simulink model "Yaw_Actuation_Testrig_org"  (Simulink 10.0)
settings: Solver=ode15s  StartTime=0.0  StopTime=40  RelTol=1e-3  EnableMultiTasking=on
undefined symbols (not defined in the file): sigbuilder_block, WT_Params
libraries: fl_lib x6, nesl_utility x3, Yaw_Motor_Lib x1, Yaw_Gearbox_Lib x1
Description:
  | Copyright 2009-2017 The MathWorks, Inc. MathWorks, Inc.
settings Model: Creator=smiller  LastModifiedBy=bhisma
settings DataIOCC: LimitDataPoints=on  SignalLoggingSaveFormat=ModelDataLogs
settings OptimizationCC: ExpressionDepthLimit=2147483647
settings DebuggingCC: FcnCallInpInsideContextMsg=warning  AllowSymbolicDim=off  StateNameClashWarn=warning
settings GRTTargetCC: GeneratePreprocessorConditionals=Disable all
settings ConfigComp: CovExternalEMLEnable=off  CovSFcnEnable=off
settings SimscapeCC: SimscapeNormalizeSystem=off  SimscapeNominalValues="[{\"value\":\"10\",\"unit\":\"V\"},{\"value\":\"1\",\"unit\":\"A\"},{\"value\":\"10\",\"unit\":\"N*m\"},{\"value\":\"10\",\"unit\":\"bar\"},{\"value\":\"100\",\"unit\":\"kJ/kg\"},{\"value\":\"1\",\"unit\":\"kW\"},{\"value\":\"300\",\"unit\":\"K\"},{\"value\":\"100\",\"unit\":\"cm^3/s\"},{\"value\":\"1\",\"unit\":\"kN\"},{\"value\":\"1\",\"unit\":\"g/cm^3\"},{\"value\":\"1\",\"unit\":\"l\"},{\"value\":\"1\",\"unit\":\"cm^2\"},{\"value\":\"60\",\"unit\":\"Hz\"}]"

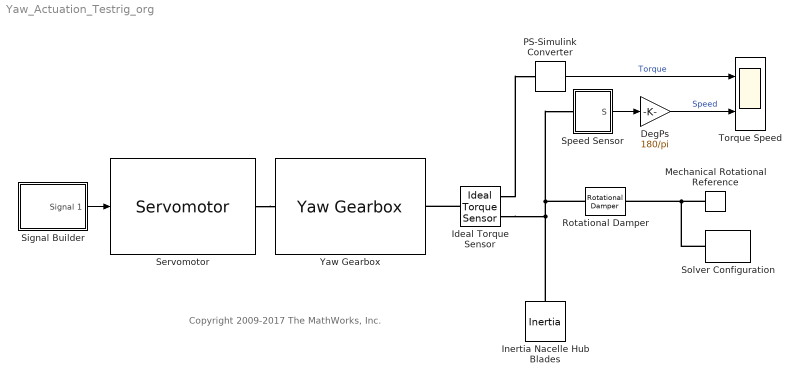
== system Yaw_Actuation_Testrig_org ==
  note: Copyright 2009-2017 The MathWorks, Inc.
  DegPs : Gain  Gain=180/pi
  Ideal Torque Sensor : fl_lib/Mechanical/Mechanical Sensors/Ideal Torque Sensor
  Inertia Nacelle Hub Blades : fl_lib/Mechanical/Rotational Elements/Inertia  inertia=WT_Params.Nacelle.inertia(1,1)*10 kg*m^2  w_specify=on  w_priority=High  w=0 rad/s  w_nominal_specify=off  w_nominal_unit=rad/s  w_nominal_value=1  t_specify=off  t_priority=High  t=0 N*m  t_nominal_specify=off  t_nominal_unit=N*m  t_nominal_value=1
  Mechanical Rotational Reference : fl_lib/Mechanical/Rotational Elements/Mechanical Rotational Reference
  PS-Simulink Converter : nesl_utility/PS-Simulink Converter  PhysicalDomain=network_engine_domain  SubClassName=ps_output  LeftPortType=input  RightPortType=output  PseudoPeriodic=off  Frequencies=[]  Unit=1  AffineConversion=off
  Rotational Damper : fl_lib/Mechanical/Rotational Elements/Rotational Damper  D=WT_Params.Nacelle.damping/4 N*m/(rad/s)  w_specify=off  w_priority=High  w=0 rad/s  w_nominal_specify=off  w_nominal_unit=rad/s  w_nominal_value=1  t_specify=off  t_priority=High  t=0 N*m  t_nominal_specify=off  t_nominal_unit=N*m  t_nominal_value=1
  Servomotor : Yaw_Motor_Lib/Yaw Motor/Servomotor  SystemSampleTime=-1
  Signal Builder : Subsystem  Tag=STV Subsys  LoadFcn=sigbuilder_block('load');  StartFcn=sigbuilder_block('start');  StopFcn=sigbuilder_block('stop');  ClipboardFcn=sigbuilder_block('clipboard');  mask(Sigbuilder block){tuvar=[0:10]}
      mask help: Create and generate interchangeable groups of signals whose waveforms are piecewise linear.
      mask init:
      | if ~strcmp(get_param(bdroot(gcbh),'SimulationStatus'),'stopped') tuvar = sigbuilder_block('maskInit'); end
      settings: CopyFcn=sigbuilder_block('copy');  DeleteFcn=sigbuilder_block('delete');  ModelCloseFcn=sigbuilder_block('modelClose');  PreSaveFcn=sigbuilder_block('preSave');  PauseFcn=sigbuilder_block('pause')  ContinueFcn=sigbuilder_block('continue')  NameChangeFcn=sigbuilder_block('namechange');  OpenFcn=sigbuilder_block('open',[437.25 199.5 550.5 399.75 ]);  CloseFcn=sigbuilder_block('close');
      mask Display: plot(0, 0, 100, 100,[2, 2, 32, 32, 2], [68, 8, 8, 68, 68],[32, 2], [38, 38], [32, 19, 2],[53, 60, 44], [32, 17, 17, 2],[16, 16, 31, 31]);txt = getActiveGroup(gcbh);text(2, 100, txt,'verticalAlignment', 'top');
  Solver Configuration : nesl_utility/Solver Configuration  PhysicalDomain=network_engine_domain  SubClassName=solver  LeftPortType=input  RightPortType=generic  Tones=[]  Harmonics=[]  SimulateNoise=off  Profile=off  UseLocalSampling=off  EnableSwitchedLinearOptims=on  FrequencyDomain=off  UseCCode=off  RelTol=0.001  AbsTol=1e-06  MinStep=1e-09  ToWorkspace=off  RevertToSquareIcSolve=off  NumHomotopyIterations=100  PhasorMode=off  PhasorModeNumHarmonics=1  DoDC=off  ResidualTolerance=1e-9  UseLocalSolver=off  LocalSolverChoice=NE_BACKWARD_EULER_ADVANCER  LocalSolverSampleTime=.001  DoFixedCost=off  MaxNonlinIter=3  MaxModeIter=2  LinearAlgebra=Sparse  EquationFormulation=NE_TIME_EF  DelaysMemoryBudget=1024  AutomaticFiltering=on  FilteringTimeConstant=0.001  PartitionStorageMethod=AS_NEEDED  PartitionMemoryBudget=1024  PartitionMethod=FAST
  Speed Sensor : Subsystem
      mask Display:
      | plot([149.600878633536;150.016472378793;150.47508104106;150.972287968219;151.50330478576;152.063017511447;152.646035805762;153.246744883819;153.859359588817;154.477980106257;155.096648782383;155.709407499646;156.310355056631;156.893703999851;157.453836360095;157.985357756531;158.483149347555;158.942417128023;159.358738098149;159.728102859405;160.046954227227;160.312221488639;160.521349974904;160.672325664379;160.763694578642;160.794576785101;160.764674871227;160.674276808796;160.524253180566;160.316048796087;160.051668777399;159.733659248606;159.365082815313;158.949489070056;158.490880407788;157.993673480629;157.462656663088;156.908284800231], [156.971389291536;157.430657072004;157.84697804213;158.216342803387;158.535194171208;158.80046143262;159.009589918885;159.16056560836;159.251934522623;159.282816729083;159.252914815208;159.162516752777;159.012493124547;158.804288740068;158.53990872138;158.221899192587;157.853322759294;157.437729014037;156.979120351769;156.48191342461;155.950896607069;155.391183881382;154.808165587067;154.20745650901;153.594841804012;152.976221286573;152.357552610446;151.744793893183;151.143846336199;150.560497392978;150.000365032735;149.468843636298;148.971052045274;148.511784264806;148.095463294681;147.726098533424;147.407247165603;147.144199990631])
      | plot([152.057635404444;152.93604260309;153.834625296826;154.744729643097;155.657590839533;156.564417533794;157.45647648909;158.325176690034;159.162152078811;159.959342124889;160.709069452336;161.404113777147;162.037781442523;162.603969882449;163.097226392739;163.512800643557;163.846690427691;164.095680203997;164.257372064819;164.330208829146;164.313489039122;164.27939575172], [142.228020686971;141.979030910664;141.817339049842;141.744502285515;141.761222075539;141.867337399197;142.061826307913;142.342815767178;142.707599694895;143.152665022428;143.673725527376;144.265763112236;144.923076131425;145.639334301243;146.40763966397;147.220593018964;148.070365181011;148.948772379657;149.847355073393;150.757459419663;151.6703206161;152.055850472277])
      | plot([116.468514315784;116.438789536125;116.349901463023;116.202706137216;115.998621130155;115.739611892022;115.42817282337;115.067303252679;114.660478551187;114.211616663162;113.725040373958;113.205435679231;112.657806656235;112.087427271827;111.499790591278;110.900555877058;110.29549408704;109.690432297022;109.091197582803;108.503560902254;107.933181517846;107.38555249485;106.865947800123;106.379371510919;105.930509622894;105.523684921402;105.162815350711;104.851376282059;104.592367043926;104.388282036865;104.241086711057;104.152198637956;104.122473858297;104.152198637956;104.241086711057;104.388282036865;104.592367043926;104.851376282059;105.162815350711;105.523684921402;105.930509622894;106.379371510919;106.865947800123;107.38555249485;107.933181517846;108.503560902254;109.091197582803;109.690432297022;110.29549408704;110.900555877058;111.499790591278;112.087427271827;112.657806656235;113.205435679231;113.725040373958;114.211616663162;114.660478551187;115.067303252679;115.42817282337;115.739611892022;115.998621130155;116.202706137216;116.349901463023;116.438789536125;116.468514315784;116.468514315784], [111.618284136057;111.013222346039;110.413987631819;109.826350951271;109.255971566862;108.708342543866;108.188737849139;107.702161559936;107.253299671911;106.846474970419;106.485605399728;106.174166331075;105.915157092943;105.711072085881;105.563876760074;105.474988686973;105.445263907313;105.474988686973;105.563876760074;105.711072085881;105.915157092943;106.174166331075;106.485605399728;106.846474970419;107.253299671911;107.702161559936;108.188737849139;108.708342543866;109.255971566862;109.826350951271;110.413987631819;111.013222346039;111.618284136057;112.223345926075;112.822580640295;113.410217320843;113.980596705252;114.528225728247;115.047830422975;115.534406712178;115.983268600203;116.390093301695;116.750962872386;117.062401941038;117.321411179171;117.525496186232;117.67269151204;117.761579585141;117.7913043648;117.761579585141;117.67269151204;117.525496186232;117.321411179171;117.062401941038;116.750962872386;116.390093301695;115.983268600203;115.534406712178;115.047830422975;114.528225728247;113.980596705252;113.410217320843;112.822580640295;112.223345926075;111.618284136057;111.618284136057])
      | plot([239.23602886498;238.828071429858;237.608127977604;235.587947230552;232.78698463364;229.232214987837;224.957872668068;220.005121927465;214.421660463109;208.261260061133;201.583248745024;194.451939414329;186.936010476274;179.107844435155;171.042830809261;162.818640088593;154.514475725591;146.210311362589;137.986120641921;129.921107016027;122.092940974909;114.577012036853;107.445702706158;100.76769139005;94.607290988073;89.0238295237172;84.0710787831142;79.7967364633452;76.2419668175427;73.4410042206305;71.4208234735788;70.2008800213248;69.7929225862026;70.2008800213248;71.4208234735788;73.4410042206306;76.2419668175428;79.7967364633454;84.0710787831144;89.0238295237174;94.6072909880733;100.76769139005;107.445702706159;114.577012036853;122.092940974909;129.921107016027;137.986120641921;146.210311362589;154.514475725591;162.818640088593;171.042830809261;179.107844435155;186.936010476274;194.451939414329;201.583248745024;208.261260061133;214.421660463109;220.005121927465;224.957872668068;229.232214987837;232.78698463364;235.587947230552;237.608127977604;238.828071429858;239.23602886498;239.23602886498], [155.774275772274;147.47628550917;139.258209428443;131.199192095207;123.376846251889;115.866505365088;108.740498123116;102.067451871182;95.9116316925529;90.3323215006612;85.3832531026163;81.1120887325275;77.5599620381344;74.7610819412943;72.742403187363;71.5233667562631;71.1157126352191;71.5233667562631;72.742403187363;74.7610819412943;77.5599620381345;81.1120887325275;85.3832531026164;90.3323215006612;95.9116316925529;102.067451871182;108.740498123116;115.866505365089;123.376846251889;131.199192095207;139.258209428443;147.47628550917;155.774275772274;164.072266035377;172.290342116104;180.34935944934;188.171705292658;195.682046179459;202.808053421432;209.481099673365;215.636919851994;221.216230043886;226.165298441931;230.43646281202;233.988589506413;236.787469603253;238.806148357184;240.025184788284;240.432838909328;240.025184788284;238.806148357184;236.787469603253;233.988589506413;230.43646281202;226.165298441931;221.216230043886;215.636919851994;209.481099673365;202.808053421432;195.682046179459;188.171705292658;180.34935944934;172.290342116105;164.072266035378;155.774275772274;155.774275772274])
      | plot([252.715889364481;252.243022716633;250.828976737403;248.487369462568;245.240751850236;241.120390602797;236.165967051481;230.425195003451;223.953361231755;216.812793033479;209.072257983804;200.806301666664;192.094529760025;183.020841389688;173.672621134841;164.139897466795;154.514475725591;144.889053984387;135.356330316341;126.008110061494;116.934421691157;108.222649784518;99.9566934673787;92.2161584177032;85.075590219427;78.6037564477313;72.8629843997015;67.9085608483856;63.7881996009461;60.5415819886144;58.199974713779;56.7859287345493;56.3130620867014;56.7859287345493;58.1999747137791;60.5415819886146;63.7881996009463;67.9085608483858;72.8629843997018;78.6037564477315;85.0755902194273;92.2161584177035;99.9566934673791;108.222649784519;116.934421691157;126.008110061494;135.356330316341;144.889053984387;154.514475725591;164.139897466796;173.672621134841;183.020841389688;192.094529760025;200.806301666664;209.072257983803;216.812793033479;223.953361231755;230.425195003451;236.165967051481;241.120390602797;245.240751850236;248.487369462568;250.828976737403;252.243022716633;252.715889364481;252.715889364481], [154.514475725591;144.895228084285;135.36861905618;126.026395093992;116.958526921455;108.252343066071;99.9916888376535;92.2561188521535;85.1201308772245;78.6524483779929;72.9153586725213;67.9641130708855;63.8463947748555;60.6018596625959;58.2617543808809;56.8486154228053;56.3760520890355;56.8486154228053;58.2617543808809;60.6018596625959;63.8463947748555;67.9641130708856;72.9153586725213;78.652448377993;85.1201308772246;92.2561188521536;99.9916888376536;108.252343066072;116.958526921455;126.026395093992;135.36861905618;144.895228084285;154.514475725591;164.133723366898;173.660332395002;183.002556357191;192.070424529728;200.776608385111;209.037262613529;216.772832599029;223.908820573958;230.37650307319;236.113592778661;241.064838380297;245.182556676327;248.427091788587;250.767197070302;252.180336028377;252.652899362147;252.180336028377;250.767197070301;248.427091788587;245.182556676327;241.064838380297;236.113592778661;230.37650307319;223.908820573958;216.772832599029;209.037262613529;200.776608385111;192.070424529728;183.002556357191;173.660332395002;164.133723366898;154.514475725592;154.514475725591])
      | plot([154.514475725591;129.948374815285;179.017586633563;154.514475725591], [240.369848906994;203.583687543869;203.583687543869;240.369848906994])
      | plot([105.382273904979;149.60125554353], [115.271704271436;156.971085816622])
      | plot([144.688035361469;144.688035361469], [152.057865634561;203.583687543869])
      | plot([164.277926087379;164.277926087379], [152.057865634561;203.583687543869])
      | plot([159.112745895982;159.616665914655], [149.60125554353;149.60125554353])
      | plot([115.208714269102;159.364705905318], [107.901873998344;149.60125554353])
      | plot([0;311.800511553884;311.800511553884;0;0], [311.800511553884;311.800511553884;0;0;311.800511553884])
      | ;
      | color('red');
      | port_label('LConn', 1,'R')
      | port_label('output', 1,'W')
  Torque Speed : Scope  NumInputPorts=2
  Yaw Gearbox : Yaw_Gearbox_Lib/Yaw Gearbox  SystemSampleTime=-1
  wires:
  Signal Builder/1(Signal 1) -> Servomotor/1
  Speed Sensor/1(S) -> DegPs/1
  PS-Simulink Converter/1 -> Torque Speed/1  "Torque"
  DegPs/1 -> Torque Speed/2  "Speed"
  connections:
  Ideal Torque Sensor/RConn1 -- Speed Sensor/LConn1 -- Rotational Damper/LConn1 -- Inertia Nacelle Hub Blades/LConn1
  Mechanical Rotational Reference/LConn1 -- Solver Configuration/RConn1 -- Rotational Damper/RConn1
  Ideal Torque Sensor/LConn1 -- Yaw Gearbox/RConn1
  Ideal Torque Sensor/RConn2 -- PS-Simulink Converter/LConn1
  Servomotor/RConn1 -- Yaw Gearbox/LConn1

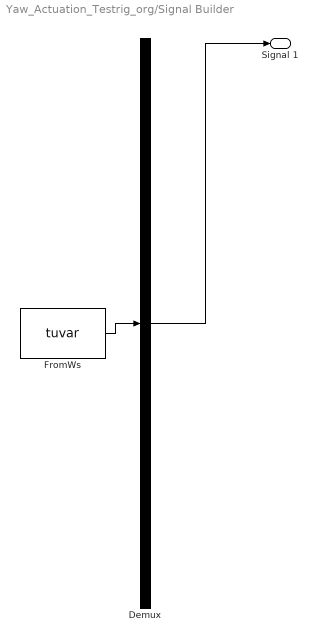
== system Yaw_Actuation_Testrig_org/Signal Builder ==
  Demux : Demux  Tag=STV Demux  Outputs=1
  FromWs : FromWorkspace  Tag=STV FromWs  VariableName=tuvar  SampleTime=0  SigBuilderData=DataTag0  VnvData=DataTag1
      SigBuilderData=|
      | common.afterFinalStr = 'Extrapolate'
      | common.sampleTime = 0
      | dataSet.timeRange = [0 40]
      | dataSet.name = 'Group 1'
      | sbobj.Groups.Name = 'Group 1'
      | sbobj.Groups.Signals.Name = 'Signal 1'
      | sbobj.Groups.Signals.XData = [0 2 5 10 15 20 24.8 28.8 32.4 40]
      | sbobj.Groups.Signals.YData = [0 0 45 45 0 0 -45 -45 0 0]
      | sbobj.Groups.TimeRange = [0 40]
  Signal 1 : Outport  Tag=STV Outport
  wires:
  Demux/1 -> Signal 1/1
  FromWs/1 -> Demux/1

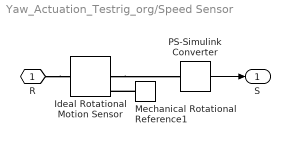
== system Yaw_Actuation_Testrig_org/Speed Sensor ==
  Ideal Rotational Motion Sensor : fl_lib/Mechanical/Mechanical Sensors/Ideal Rotational Motion Sensor  offset=0 rad
  Mechanical Rotational Reference1 : fl_lib/Mechanical/Rotational Elements/Mechanical Rotational Reference
  PS-Simulink Converter : nesl_utility/PS-Simulink Converter  PhysicalDomain=network_engine_domain  SubClassName=ps_output  LeftPortType=input  RightPortType=output  PseudoPeriodic=off  Frequencies=[]  Unit=1  AffineConversion=off
  R : PMIOPort  Side=Left
  S : Outport
  wires:
  PS-Simulink Converter/1 -> S/1
  connections:
  Ideal Rotational Motion Sensor/RConn2 -- PS-Simulink Converter/LConn1
  R/RConn1 -- Ideal Rotational Motion Sensor/LConn1
  Mechanical Rotational Reference1/LConn1 -- Ideal Rotational Motion Sensor/RConn1
